simulink model "Susp_system"  (R2020a)
settings: Solver=VariableStepAuto  StartTime=0.0  StopTime=100  RelTol=1e-3
settings Model: Creator=DELL  LastModifiedBy=DELL

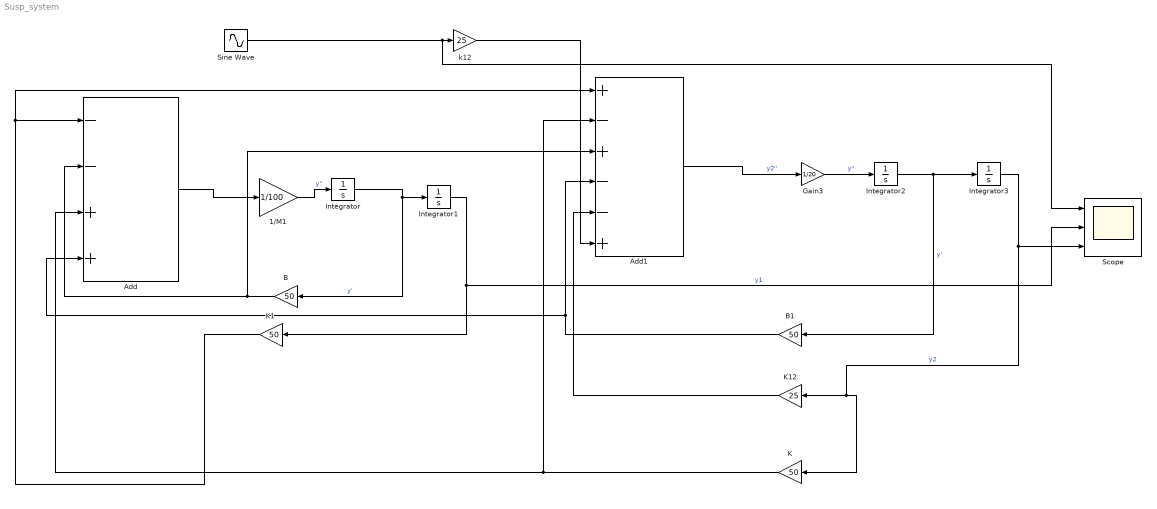
== system Susp_system ==
  1/M1 : Gain  Gain=1/100
  Add : Sum  Inputs=--++
  Add1 : Sum  Inputs=+-+--+
  B : Gain  Gain=50
  B1 : Gain  Gain=50
  Gain3 : Gain  Gain=1/20
  Integrator{,1..3} (4 alike) : Integrator
  K : Gain  Gain=50
  K1 : Gain  Gain=50
  K12 : Gain  Gain=25
  Scope : Scope  NumInputPorts=3
  Sine Wave : Sin  Amplitude=2  Frequency=10  SampleTime=0
  k12 : Gain  Gain=25
  wires:
  Add/1 -> 1/M1/1
  1/M1/1 -> Integrator/1  "y''"
  Integrator/1 -> Integrator1/1, B/1  "y'"
  Integrator1/1 -> K1/1, Scope/2  "y1"
  K1/1 -> Add1/1, Add/1
  B/1 -> Add1/3, Add/2
  Add1/1 -> Gain3/1  "y2''"
  Gain3/1 -> Integrator2/1  "y''"
  Integrator2/1 -> B1/1, Integrator3/1  "y'"
  Integrator3/1 -> K12/1, K/1, Scope/3  "y2"
  K/1 -> Add/3, Add1/2
  B1/1 -> Add/4, Add1/4
  K12/1 -> Add1/5
  Sine Wave/1 -> Scope/1, k12/1
  k12/1 -> Add1/6
